simulink model "matlab_function_code_trial"  (R2018b)
settings: Solver=VariableStepAuto  StartTime=0.0  StopTime=10.0  RelTol=1e-3
settings Model: Creator=marwan  LastModifiedBy=marwan

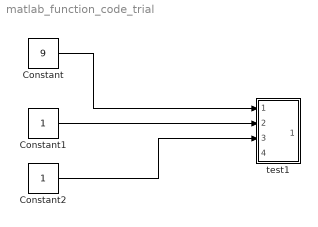
== system matlab_function_code_trial ==
  Constant : Constant  Value=9
  Constant1 : Constant
  Constant2 : Constant
  test1 : Subsystem  mask{Parameter1=0, Parameter2=0}
  wires:
  Constant/1 -> test1/1(In1)
  Constant1/1 -> test1/2(In2)
  Constant2/1 -> test1/3(In3)

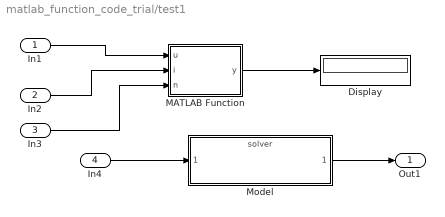
== system matlab_function_code_trial/test1 ==
  In1 : Inport
  In2 : Inport  Port=2
  In3 : Inport  Port=3
  In4 : Inport  Port=4
  Display : Display
  MATLAB Function : MATLAB Function  TreatAsAtomicUnit=on
  Model : ModelReference  ModelNameDialog=solver.slx  SimulationMode=Normal  ModelReferenceVersion=1.8
  Out1 : Outport
  wires:
  In2/1 -> MATLAB Function/2(i)
  In4/1 -> Model/1
  Model/1 -> Out1/1
  In1/1 -> MATLAB Function/1(u)
  In3/1 -> MATLAB Function/3(n)
  MATLAB Function/1(y) -> Display/1

== matlab function matlab_function_code_trial/test1/MATLAB Function ==
  data: u input; y output; i input; n input
function y = fcn(u,i,n)


y = u*2+i*3-n;
